simulink model "digital_tracking_2017a"  (R2017a)
settings: Solver=ode45  StartTime=0.0  StopTime=32  RelTol=1e-3  EnableMultiTasking=on
values from neighbouring files (symbols this model uses):
  A = plant_linear_A    [design_digital.m]
  B = plant_linear_B    [design_digital.m]
  C = [1 0 0 0 0 0;0 0 0 0 1 0]    [design_digital.m]
  gammaa = eye(2)    [design_digital.m]
  K1 = Kd(:,1:6)    [design_digital.m]
  K2 = Kd(:,7:8)    [design_digital.m]
  phia = eye(2)    [design_digital.m]
  T = 0.01    [design_digital.m]
libraries: simulink x1
settings Model: Creator=rjv  LastModifiedBy=kando
settings DataIOCC: LimitDataPoints=on  SaveFormat=Array
settings OptimizationCC: LifeSpan=inf
settings DebuggingCC: AllowSymbolicDim=off  SFUnexpectedBacktrackingDiag=warning  SFNoUnconditionalDefaultTransitionDiag=warning  SFExecutionAtInitializationDiag=none
settings HardwareCC: ProdBitPerPointer=32  ProdBitPerSizeT=32  ProdBitPerPtrDiffT=32  ProdLargestAtomicFloat=None  ProdIntDivRoundTo=Undefined  ProdEndianess=Unspecified  ProdWordSize=32  ProdHWDeviceType=32-bit Generic
settings ModelReferenceCC: PropagateSignalLabelsOutOfModel=off
settings GRTTargetCC: TargetLangStandard=C89/C90 (ANSI)  GeneratePreprocessorConditionals=Disable all
settings ConfigComp: CovMetricSettings=dw  CovHtmlReporting=on  CovSaveCumulativeToWorkspaceVar=on  CovSaveSingleToWorkspaceVar=on  CovExternalEMLEnable=off

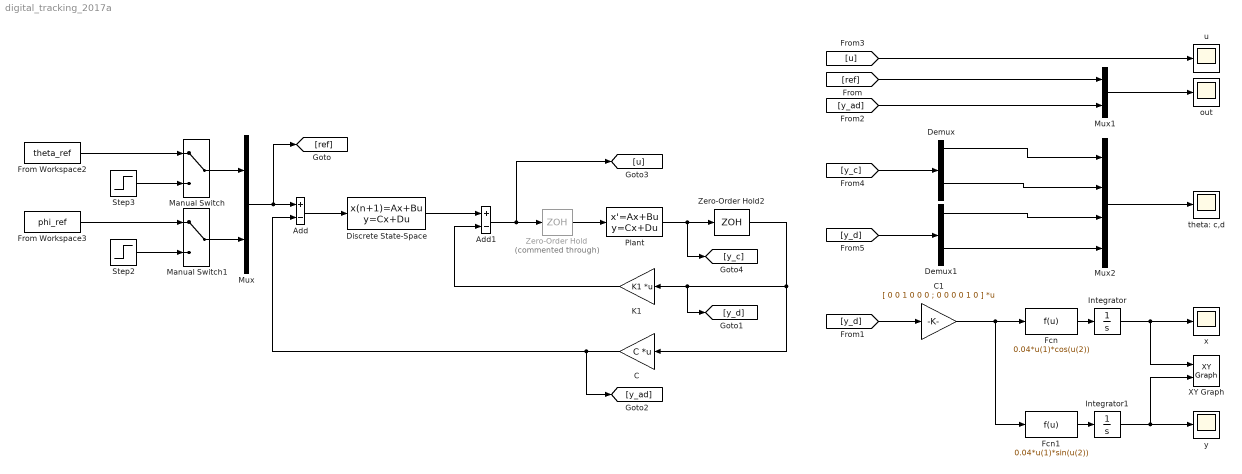
== system digital_tracking_2017a ==
  Add : Sum  Inputs=+-
  Add1 : Sum  Inputs=+-
  C : Gain  Gain=C  Multiplication=Matrix(K*u)
      settings: AttributesFormatString=%<Gain>
  C1 : Gain  Gain=[ 0 0 1 0 0 0 ; 0 0 0 0 1 0 ]  Multiplication=Matrix(K*u)
      settings: AttributesFormatString=%<Gain>
  Demux : Demux  Outputs=6
  Demux1 : Demux  Outputs=6
  Discrete State-Space : DiscreteStateSpace  A=phia  B=gammaa  C=K2  D=0*K2*gammaa  X0=K2\(K1*[0;0;0;0;pi/4;0])  SampleTime=T
  Fcn : Fcn  Expr=0.04*u(1)*cos(u(2))
  Fcn1 : Fcn  Expr=0.04*u(1)*sin(u(2))
  From Workspace2 : FromWorkspace  VariableName=theta_ref  SampleTime=0.01  OutputAfterFinalValue=Holding final value
  From Workspace3 : FromWorkspace  VariableName=phi_ref  SampleTime=0.01  OutputAfterFinalValue=Holding final value
  Integrator : Integrator
  Integrator1 : Integrator
  K1 : Gain  Gain=K1  Multiplication=Matrix(K*u)
      settings: AttributesFormatString=%<Gain>
  Manual Switch : ManualSwitch
  Manual Switch1 : ManualSwitch
  Mux : Mux  Inputs=2
  Mux1 : Mux  Inputs=2
  Mux2 : Mux
  Plant : StateSpace  A=A  B=B  C=eye(length(A))  D=zeros(length(A),min(size((B))))  X0=[0;0;0;0;0;0]
  Step2 : Step  Time=0  Before=pi/4  After=pi/4+1  SampleTime=0
  Step3 : Step  Time=0  After=5  SampleTime=0
  XY Graph : simulink/Sinks/XY Graph  xmin=-1  xmax=1  ymin=-1  ymax=1  st=-1
  Zero-Order Hold : ZeroOrderHold  Commented=through  SampleTime=T
  Zero-Order Hold2 : ZeroOrderHold  SampleTime=T
  out : Scope
  theta: c,d : Scope
  u : Scope
  x : Scope
  y : Scope
  wires:
  Add1/1 -> [u], Zero-Order Hold/1
  Discrete State-Space/1 -> Add1/1
  K1/1 -> Add1/2
  Fcn/1 -> Integrator/1
  Fcn1/1 -> Integrator1/1
  Integrator/1 -> x/1, XY Graph/1
  Integrator1/1 -> XY Graph/2, y/1
  C1/1 -> Fcn/1, Fcn1/1
  Mux1/1 -> out/1
  Mux/1 -> [ref], Add/1
  Step2/1 -> Manual Switch1/2
  From Workspace3/1 -> Manual Switch1/1
  Manual Switch1/1 -> Mux/2
  Manual Switch/1 -> Mux/1
  Step3/1 -> Manual Switch/2
  From Workspace2/1 -> Manual Switch/1
  Add/1 -> Discrete State-Space/1
  Zero-Order Hold/1 -> Plant/1
  Zero-Order Hold2/1 -> [y_d], K1/1, C/1
  [ref] -> Mux1/1
  [y_d] -> C1/1
  [y_ad] -> Mux1/2
  [u] -> u/1
  C/1 -> [y_ad], Add/2
  [y_d] -> Demux1/1
  [y_c] -> Demux/1
  Mux2/1 -> theta: c,d/1
  Demux/1 -> Mux2/1
  Demux1/1 -> Mux2/3
  Plant/1 -> [y_c], Zero-Order Hold2/1
  Demux1/5 -> Mux2/4
  Demux/5 -> Mux2/2
